simulink model "geos3"  (Simulink 5.0)
settings: Solver=ode23s  StartTime=0.0  StopTime=12000  RelTol=1e-3
undefined symbols (not defined in the file): A, B, n
libraries: simulink x2

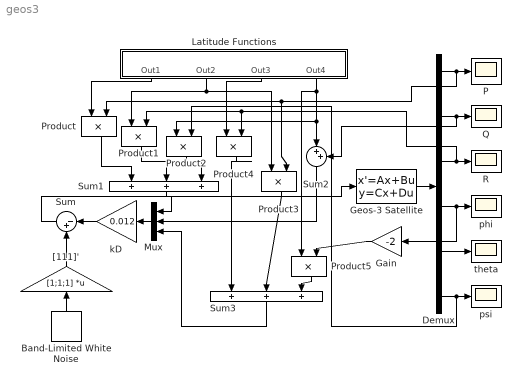
== system geos3 ==
  Band-Limited White Noise : simulink/Sources/Band-Limited White Noise  Orientation=up  Cov=[1e-10]  Ts=0.1  seed=[23341]
  Demux : Demux  Outputs=6
  Gain : Gain  Orientation=left  Gain=-2  SaturateOnIntegerOverflow=on
  Geos-3 Satellite : StateSpace  A=A  B=B  C=eye(size(A))  D=zeros(size(B))  X0=[0 0 0 0.01 0.002 0]'
  Latitude Functions : Subsystem  Orientation=down
  Mux : Mux  Orientation=left  Inputs=3
  P : Scope
      settings: SaveName=P  DataFormat=Array  MaxDataPoints=500  Decimation=100
  Product{,1..5} (6 alike) : Product  Orientation=down  SaturateOnIntegerOverflow=on
  Q : Scope
      settings: YMin=-8e-006  YMax=8e-006  SaveName=Q  DataFormat=Array  MaxDataPoints=500  Decimation=100
  R : Scope
      settings: SaveName=R  DataFormat=Array  MaxDataPoints=500  Decimation=100
  Sum : Sum  Orientation=left  Inputs=|-+  SaturateOnIntegerOverflow=on
  Sum1 : Sum  Orientation=down  Inputs=|+++  SaturateOnIntegerOverflow=on
  Sum2 : Sum  Orientation=down  Inputs=|++  SaturateOnIntegerOverflow=on
  Sum3 : Sum  Orientation=down  Inputs=|+++  SaturateOnIntegerOverflow=on
  "[111]'" : Gain  Orientation=up  Gain=[1;1;1]  Multiplication=Matrix(K*u)  SaturateOnIntegerOverflow=on
  kD : Gain  Orientation=left  Gain=0.012  SaturateOnIntegerOverflow=on
  phi : Scope
      settings: SaveName=phi  DataFormat=Array  MaxDataPoints=500  Decimation=100
  psi : Scope
      settings: SaveName=psi  DataFormat=Array  MaxDataPoints=500  Decimation=100
  theta : Scope
      settings: YMin=-0.0045  YMax=0.002  SaveName=theta  DataFormat=Array  MaxDataPoints=500  Decimation=100
  wires:
  Demux/1 -> P/1, Product/2, Product3/2
  Demux/2 -> Q/1, Sum2/2
  Demux/3 -> R/1, Product1/2, Product4/2
  Demux/4 -> phi/1, Gain/1
  Demux/5 -> theta/1
  Demux/6 -> psi/1, Product2/2
  Geos-3 Satellite/1 -> Demux/1
  Latitude Functions/2(Out2) -> Product3/1, Product1/1
  Product/1 -> Sum1/1
  Product2/1 -> Sum1/3
  Latitude Functions/4(Out4) -> Product2/1, Sum2/1, Product5/1
  Latitude Functions/3(Out3) -> Product4/1
  Gain/1 -> Product5/2
  Product5/1 -> Sum3/3
  Product3/1 -> Sum3/2
  Product4/1 -> Sum3/1
  Sum1/1 -> Mux/1
  Sum2/1 -> Mux/2
  Sum3/1 -> Mux/3
  Mux/1 -> kD/1
  kD/1 -> Sum/1
  Band-Limited White Noise/1 -> "[111]'"/1
  Sum/1 -> Geos-3 Satellite/1
  "[111]'"/1 -> Sum/2
  Product1/1 -> Sum1/2
  Latitude Functions/1(Out1) -> Product/1

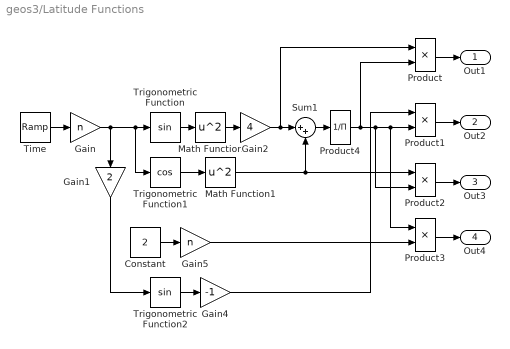
== system geos3/Latitude Functions ==
  Constant : Constant  Value=2
  Gain : Gain  Gain=n  SaturateOnIntegerOverflow=on
  Gain1 : Gain  Orientation=down  Gain=2  SaturateOnIntegerOverflow=on
  Gain2 : Gain  Gain=4  SaturateOnIntegerOverflow=on
  Gain4 : Gain  Gain=-1  SaturateOnIntegerOverflow=on
  Gain5 : Gain  Gain=n  SaturateOnIntegerOverflow=on
  Math Function : Math  Operator=square
  Math Function1 : Math  Operator=square
  Product{,1..3} (4 alike) : Product  SaturateOnIntegerOverflow=on
  Product4 : Product  Inputs=/  SaturateOnIntegerOverflow=on
  Sum1 : Sum  Inputs=|++  SaturateOnIntegerOverflow=on
  Time : simulink/Sources/Ramp  slope=1  start=0  X0=0
  Trigonometric Function : Trigonometry  OutputSignalType=real
  Trigonometric Function1 : Trigonometry  Operator=cos
  Trigonometric Function2 : Trigonometry
  Out1 : Outport
  Out2 : Outport  Port=2
  Out3 : Outport  Port=3
  Out4 : Outport  Port=4
  wires:
  Gain/1 -> Trigonometric Function1/1, Trigonometric Function/1, Gain1/1
  Gain1/1 -> Trigonometric Function2/1
  Trigonometric Function/1 -> Math Function/1
  Trigonometric Function1/1 -> Math Function1/1
  Math Function/1 -> Gain2/1
  Gain2/1 -> Sum1/1, Product/1
  Math Function1/1 -> Sum1/2, Product2/1
  Trigonometric Function2/1 -> Gain4/1
  Constant/1 -> Gain5/1
  Product/1 -> Out1/1
  Product1/1 -> Out2/1
  Product2/1 -> Out3/1
  Product3/1 -> Out4/1
  Time/1 -> Gain/1
  Gain5/1 -> Product3/2
  Sum1/1 -> Product4/1
  Product4/1 -> Product/2, Product2/2, Product1/2, Product3/1
  Gain4/1 -> Product1/1
